simulink model "SWC_FDC_type"  (R2021b)
settings: Solver=FixedStepDiscrete  StartTime=0.0  StopTime=10.0  FixedStep=0.001  RelTol=1e-3
values from neighbouring files (symbols this model uses):
  C_TASK_5MS_S = (	C_TICK_TIME_S      	)    [vcu_local_hdr.m]
  DID_VCUKey = uint16(0x0202)    [vcu_local_hdr.m]
  DID_XWD = uint16(513)    [vcu_local_hdr.m]
  DIDLen_DKCKey = uint16(8)    [vcu_local_hdr.m]
  DIDLen_FoxPiBattSta = uint16(4)    [vcu_local_hdr.m]
  DIDLen_FoxPiBrakeSta = uint16(13)    [vcu_local_hdr.m]
  DIDLen_FoxPiButtonSta = uint16(2)    [vcu_local_hdr.m]
  DIDLen_FoxPiCtrlEnSw = uint16(1)    [vcu_local_hdr.m]
  DIDLen_FoxPiDrivingCtrl = uint16(21)    [vcu_local_hdr.m]
  DIDLen_FoxPiEPSSta = uint16(11)    [vcu_local_hdr.m]
  DIDLen_FoxPiLampCtrl = uint16(6)    [vcu_local_hdr.m]
  DIDLen_FoxPiLampSta = uint16(2)    [vcu_local_hdr.m]
  DIDLen_FoxPiMotionSta = uint16(13)    [vcu_local_hdr.m]
  DIDLen_FoxPiMotorSta = uint16(11)    [vcu_local_hdr.m]
  DIDLen_FoxPiPedalPos = uint16(3)    [vcu_local_hdr.m]
  DIDLen_FoxPiPTGUSSSw = uint16(1)    [vcu_local_hdr.m]
  DIDLen_FoxPiShifterAllow = uint16(3)    [vcu_local_hdr.m]
  DIDLen_FoxPiSwSta = uint16(2)    [vcu_local_hdr.m]
  DIDLen_FoxPiTPMSSta = uint16(13)    [vcu_local_hdr.m]
  DIDLen_FoxPiUSSDist = uint16(20)    [vcu_local_hdr.m]
  DIDLen_FoxPiUSSFaultSta = uint16(2)    [vcu_local_hdr.m]
  DIDLen_FoxPiWheelSpd = uint16(16)    [vcu_local_hdr.m]
  DIDNum_DKCKey = uint16(0x0202)    [vcu_local_hdr.m]
  DIDNum_FoxPiBattSta = uint16(0x100D)    [vcu_local_hdr.m]
  DIDNum_FoxPiBrakeSta = uint16(0x1003)    [vcu_local_hdr.m]
  DIDNum_FoxPiButtonSta = uint16(0x1006)    [vcu_local_hdr.m]
  DIDNum_FoxPiCtrlEnSw = uint16(0x1012)    [vcu_local_hdr.m]
  DIDNum_FoxPiDrivingCtrl = uint16(0x1001)    [vcu_local_hdr.m]
  DIDNum_FoxPiEPSSta = uint16(0x1005)    [vcu_local_hdr.m]
  DIDNum_FoxPiLampCtrl = uint16(0x100C)    [vcu_local_hdr.m]
  DIDNum_FoxPiLampSta = uint16(0x100B)    [vcu_local_hdr.m]
  DIDNum_FoxPiMotionSta = uint16(0x1002)    [vcu_local_hdr.m]
  DIDNum_FoxPiMotorSta = uint16(0x1010)    [vcu_local_hdr.m]
  DIDNum_FoxPiPedalPos = uint16(0x100F)    [vcu_local_hdr.m]
  DIDNum_FoxPiPTGUSSSw = uint16(0x1009)    [vcu_local_hdr.m]
  DIDNum_FoxPiShifterAllow = uint16(0x1011)    [vcu_local_hdr.m]
  DIDNum_FoxPiSwSta = uint16(0x100A)    [vcu_local_hdr.m]
  DIDNum_FoxPiTPMSSta = uint16(0x100E)    [vcu_local_hdr.m]
  DIDNum_FoxPiUSSDist = uint16(0x1007)    [vcu_local_hdr.m]
  DIDNum_FoxPiUSSFaultSta = uint16(0x1008)    [vcu_local_hdr.m]
  DIDNum_FoxPiWheelSpd = uint16(0x1004)    [vcu_local_hdr.m]
  DIDVCUKeyLength = uint16(8)    [vcu_local_hdr.m]
  DTC_10020B = Simulink.Parameter    [DTC_Constant_Definition.m]
  DTC_10020C = Simulink.Parameter    [DTC_Constant_Definition.m]
  DTC_10020D = Simulink.Parameter    [DTC_Constant_Definition.m]
  DTC_10020E = Simulink.Parameter    [DTC_Constant_Definition.m]
  DTC_100210 = Simulink.Parameter    [DTC_Constant_Definition.m]
  DTC_100211 = Simulink.Parameter    [DTC_Constant_Definition.m]
  DTC_100212 = Simulink.Parameter    [DTC_Constant_Definition.m]
  DTC_100213 = Simulink.Parameter    [DTC_Constant_Definition.m]
  DTC_100214 = Simulink.Parameter    [DTC_Constant_Definition.m]
  DTC_100215 = Simulink.Parameter    [DTC_Constant_Definition.m]
  DTC_100216 = Simulink.Parameter    [DTC_Constant_Definition.m]
  DTC_100217 = Simulink.Parameter    [DTC_Constant_Definition.m]
  DTC_100218 = Simulink.Parameter    [DTC_Constant_Definition.m]
  DTC_100219 = Simulink.Parameter    [DTC_Constant_Definition.m]
  DTC_10021A = Simulink.Parameter    [DTC_Constant_Definition.m]
  DTC_10021B = Simulink.Parameter    [DTC_Constant_Definition.m]
  DTC_10021C = Simulink.Parameter    [DTC_Constant_Definition.m]
  DTC_10021D = Simulink.Parameter    [DTC_Constant_Definition.m]
  DTC_10021E = Simulink.Parameter    [DTC_Constant_Definition.m]
  DTC_100220 = Simulink.Parameter    [DTC_Constant_Definition.m]
  DTC_100221 = Simulink.Parameter    [DTC_Constant_Definition.m]
  DTC_100223 = Simulink.Parameter    [DTC_Constant_Definition.m]
  DTC_100224 = Simulink.Parameter    [DTC_Constant_Definition.m]
  DTC_100225 = Simulink.Parameter    [DTC_Constant_Definition.m]
  DTC_100226 = Simulink.Parameter    [DTC_Constant_Definition.m]
  DTC_100227 = Simulink.Parameter    [DTC_Constant_Definition.m]
  DTC_100242 = Simulink.Parameter    [DTC_Constant_Definition.m]
  DTC_100243 = Simulink.Parameter    [DTC_Constant_Definition.m]
  DTC_100244 = Simulink.Parameter    [DTC_Constant_Definition.m]
  DTC_100247 = Simulink.Parameter    [DTC_Constant_Definition.m]
  DTC_100248 = Simulink.Parameter    [DTC_Constant_Definition.m]
  DTC_100249 = Simulink.Parameter    [DTC_Constant_Definition.m]
  DTC_100250 = Simulink.Parameter    [DTC_Constant_Definition.m]
  DTC_100251 = Simulink.Parameter    [DTC_Constant_Definition.m]
  DTC_100252 = Simulink.Parameter    [DTC_Constant_Definition.m]
  DTC_100A10 = Simulink.Parameter    [DTC_Constant_Definition.m]
  DTC_100A12 = Simulink.Parameter    [DTC_Constant_Definition.m]
  DTC_100A16 = Simulink.Parameter    [DTC_Constant_Definition.m]
  DTC_100A17 = Simulink.Parameter    [DTC_Constant_Definition.m]
  DTC_100A18 = Simulink.Parameter    [DTC_Constant_Definition.m]
  DTC_100A19 = Simulink.Parameter    [DTC_Constant_Definition.m]
  DTC_500B01 = Simulink.Parameter    [DTC_Constant_Definition.m]
  DTC_500B02 = Simulink.Parameter    [DTC_Constant_Definition.m]
  DTC_500B03 = Simulink.Parameter    [DTC_Constant_Definition.m]
  DTC_500B04 = Simulink.Parameter    [DTC_Constant_Definition.m]
  DTC_500B05 = Simulink.Parameter    [DTC_Constant_Definition.m]
  DTC_500B06 = Simulink.Parameter    [DTC_Constant_Definition.m]
  DTC_500B07 = Simulink.Parameter    [DTC_Constant_Definition.m]
  DTC_500B08 = Simulink.Parameter    [DTC_Constant_Definition.m]
  DTC_500B09 = Simulink.Parameter    [DTC_Constant_Definition.m]
  DTC_500B0A = Simulink.Parameter    [DTC_Constant_Definition.m]
  DTC_500B0B = Simulink.Parameter    [DTC_Constant_Definition.m]
  DTC_500B0C = Simulink.Parameter    [DTC_Constant_Definition.m]
  DTC_500B0D = Simulink.Parameter    [DTC_Constant_Definition.m]
  DTC_500B0E = Simulink.Parameter    [DTC_Constant_Definition.m]
  DTC_500B0F = Simulink.Parameter    [DTC_Constant_Definition.m]
  DTC_500B10 = Simulink.Parameter    [DTC_Constant_Definition.m]
  DTC_90021F = Simulink.Parameter    [DTC_Constant_Definition.m]
  DTC_90022F = Simulink.Parameter    [DTC_Constant_Definition.m]
  DTC_900253 = Simulink.Parameter    [DTC_Constant_Definition.m]
  DTC_900254 = Simulink.Parameter    [DTC_Constant_Definition.m]
  DTC_900301 = Simulink.Parameter    [DTC_Constant_Definition.m]
  DTC_900302 = Simulink.Parameter    [DTC_Constant_Definition.m]
  DTC_900303 = Simulink.Parameter    [DTC_Constant_Definition.m]
  DTC_900304 = Simulink.Parameter    [DTC_Constant_Definition.m]
  DTC_900305 = Simulink.Parameter    [DTC_Constant_Definition.m]
  DTC_900909 = Simulink.Parameter    [DTC_Constant_Definition.m]
  DTC_90090A = Simulink.Parameter    [DTC_Constant_Definition.m]
  DTC_90090B = Simulink.Parameter    [DTC_Constant_Definition.m]
  DTC_90090C = Simulink.Parameter    [DTC_Constant_Definition.m]
  DTC_90090D = Simulink.Parameter    [DTC_Constant_Definition.m]
  DTC_90090E = Simulink.Parameter    [DTC_Constant_Definition.m]
  DTC_90090F = Simulink.Parameter    [DTC_Constant_Definition.m]
  DTC_900910 = Simulink.Parameter    [DTC_Constant_Definition.m]
  DTC_900911 = Simulink.Parameter    [DTC_Constant_Definition.m]
  DTC_900912 = Simulink.Parameter    [DTC_Constant_Definition.m]
  DTC_900913 = Simulink.Parameter    [DTC_Constant_Definition.m]
  DTC_900914 = Simulink.Parameter    [DTC_Constant_Definition.m]
  ... (+54 more)
undefined symbols (not defined in the file or in its folder): f32_ApsOutVehSpdSig, KHAL_CANBusOffDebounce_cnt, KHAL_CANBusOffDebounce_s, KHAL_DKCDecryptEnable_flg_ovrdflg, KHAL_DKCDecryptEnable_flg_ovrdval, KHAL_RandomNumberY1_enum, KHAL_RandomNumberY2_enum, KHAL_RandomNumberY_ovrdflg, KHAL_TPMSRESBUTT_flg_ovrdflg, KHAL_TPMSRESBUTT_flg_ovrdval, KINP_ReadVinCode_flg, P_boolean, R_DIDWriteCDD_CSOP_DIDSet_DKCKey, R_DIDWriteCDD_CSOP_DIDSet_FoxPiBattSta, R_DIDWriteCDD_CSOP_DIDSet_FoxPiBrakeSta, R_DIDWriteCDD_CSOP_DIDSet_FoxPiButtonSta, R_DIDWriteCDD_CSOP_DIDSet_FoxPiCtrlEnSw, R_DIDWriteCDD_CSOP_DIDSet_FoxPiDrivingCtrl, R_DIDWriteCDD_CSOP_DIDSet_FoxPiEPSSta, R_DIDWriteCDD_CSOP_DIDSet_FoxPiLampCtrl, R_DIDWriteCDD_CSOP_DIDSet_FoxPiLampSta, R_DIDWriteCDD_CSOP_DIDSet_FoxPiMotionSta, R_DIDWriteCDD_CSOP_DIDSet_FoxPiMotorSta, R_DIDWriteCDD_CSOP_DIDSet_FoxPiPedalPos, R_DIDWriteCDD_CSOP_DIDSet_FoxPiPTGUSSSw, R_DIDWriteCDD_CSOP_DIDSet_FoxPiShifterAllow, R_DIDWriteCDD_CSOP_DIDSet_FoxPiSwSta, R_DIDWriteCDD_CSOP_DIDSet_FoxPiTPMSSta, R_DIDWriteCDD_CSOP_DIDSet_FoxPiUSSDist, R_DIDWriteCDD_CSOP_DIDSet_FoxPiUSSFaultSta, R_DIDWriteCDD_CSOP_DIDSet_FoxPiWheelSpd, R_E2E_CAN3_VCU1_CSOP_Write_CAN3_VCU1, R_E2E_CAN3_VCU1_toNIDEC_CSOP_Write_CAN3_VCU1_toNIDEC, R_E2E_CAN4_VCU1_CSOP_Write_CAN4_VCU1, R_FDCCDD_Inner_CSOP_FDC_AppCallSleep, R_HALIN_IMU_CSOP_IMUSetSta, R_HALINCDD_CSOP_PAS_Handler, R_HALINCDD_CSOP_ResetPedalZeroPosDone, R_HALINCDD_CSOP_TPMSSensorIDRegSetResults, R_HALINCDD_CSOP_UDS_Main, R_HALOUT_APS_CSOP_ApsOutput, R_HALOUTCDD_CSOP_AppNmStateReq, R_HALOUTCDD_CSOP_IVIReset, R_HALOUTCDD_CSOP_SetAcoreRebootCmdACK, R_HALOUTCDD_CSOP_SetSysPwrStat ... (+80)
libraries: FVT_lib x447, simulink x289, hcu_lib x19, hdlsllib x9, app x1, halin x1, halout x1, matrix_library x1, inp x1, outp x1
(part 2 of 15)

== system SWC_FDC_type/run_SWC_FDC_PAS_1ms_sys ==
  function : TriggerPort  TriggerType=function-call  VariantControl=(inherit)  SampleTimeType=periodic  SampleTime=-1
  R_HALINCDD_CSOP_PAS_Handler : FunctionCaller  FunctionPrototype=R_HALINCDD_CSOP_PAS_Handler()
